simulink model "gm_lms"  (R2024a)
settings: Solver=FixedStepDiscrete  StartTime=0.0  StopTime=(samples-1)/fs  RelTol=1e-3  EnableMultiTasking=on
InitFcn:
  | setup;
undefined symbols (not defined in the file or in its folder): fs
libraries: dspadpt3 x1, dspsrcs4 x1
settings Model: Creator=ross  LastModifiedBy=ADMIN
settings SolverCC: AlgebraicLoopSolver=TrustRegion
settings DataIOCC: LimitDataPoints=on  SaveFormat=Array  SignalLogging=off  ReturnWorkspaceOutputs=off
settings OptimizationCC: BlockReduction=off  ConditionallyExecuteInputs=off  DefaultParameterBehavior=Inlined  LifeSpan=inf
settings DebuggingCC: AlgebraicLoopMsg=error  UnderspecifiedInitializationDetection=Classic  MergeDetectMultiDrivingBlocksExec=none  SolverPrmCheckMsg=warning  InheritedTsInSrcMsg=none  Int32ToFloatConvMsg=none  UnconnectedInputMsg=warning  UnconnectedOutputMsg=warning  UnconnectedLineMsg=warning  StateNameClashWarn=warning  SFUnexpectedBacktrackingDiag=warning  SFNoUnconditionalDefaultTransitionDiag=warning  SFExecutionAtInitializationDiag=none  ArithmeticOperatorsInVariantConditions=warning
settings HardwareCC: ProdBitPerPointer=32  ProdBitPerSizeT=32  ProdBitPerPtrDiffT=32  ProdLargestAtomicFloat=None  ProdIntDivRoundTo=Undefined  ProdEndianess=Unspecified  ProdWordSize=32  ProdHWDeviceType=ASIC/FPGA->ASIC/FPGA  ProdEqTarget=off
settings ModelReferenceCC: PropagateSignalLabelsOutOfModel=off
settings SFSimCC: SimUseLocalCustomCode=off  CustomCodeUndefinedFunction=UseInterfaceOnly
settings RTWCC: GenerateReport=on  RTWUseLocalCustomCode=off  GPUComputeCapability=3.5
settings CodeAppCC: StateflowObjectComments=on
settings GRTTargetCC: TargetLangStandard=C89/C90 (ANSI)
settings ConfigComp: CovMetricSettings=dw  CovSaveCumulativeToWorkspaceVar=on  CovSaveSingleToWorkspaceVar=on  CovExternalEMLEnable=off

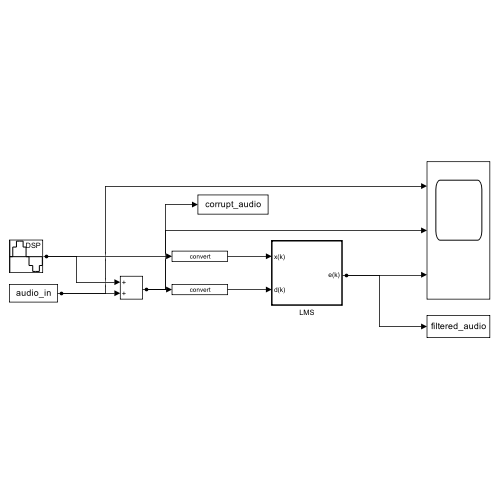
[thumbnail: Simulink's stored preview of the top-level diagram]
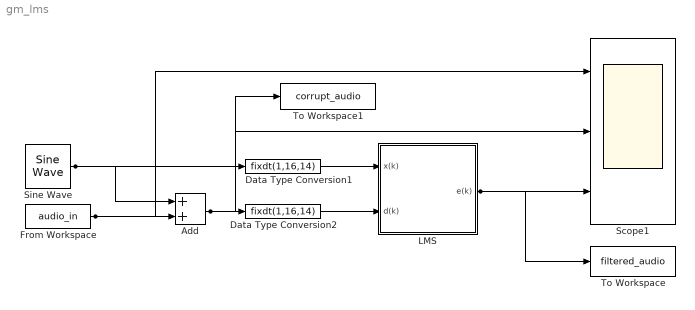
== system gm_lms ==
  Add : Sum
  Data Type Conversion1 : DataTypeConversion  OutDataTypeStr=fixdt(1,16,14)  SaturateOnIntegerOverflow=off  RndMeth=Floor
  Data Type Conversion2 : DataTypeConversion  OutDataTypeStr=fixdt(1,16,14)  SaturateOnIntegerOverflow=off  RndMeth=Floor
  From Workspace : FromWorkspace  VariableName=audio_in  SampleTime=1/fs  Interpolate=off  ZeroCross=off  OutputAfterFinalValue=Holding final value
  LMS : Subsystem  TreatAsAtomicUnit=on
  Scope1 : Scope  NumInputPorts=3
  Sine Wave : dspsrcs4/Sine Wave  Amplitude=0.75  Frequency=0.25*fs  Phase=0  SampleMode=Discrete  OutComplex=Real  CompMethod=Table lookup  TableSize=Speed  SampleTime=1/fs  SamplesPerFrame=1  ResetState=Restart at time zero  OutputFrames=on  dataType=Fixed-point  wordLen=16  udDataType=sfix(16)  fracBitsMode=User-defined  numFracBits=14  OutDataTypeStr=fixdt(1,16,14)  LastOutDataTypeStr=fixdt(1,16,14)
  To Workspace : ToWorkspace  VariableName=filtered_audio  SampleTime=-1
  To Workspace1 : ToWorkspace  VariableName=corrupt_audio  SampleTime=-1
  wires:
  Data Type Conversion2/1 -> LMS/2(d(k))
  Data Type Conversion1/1 -> LMS/1(x(k))
  LMS/1(e(k)) -> Scope1/3, To Workspace/1
  Add/1 -> Scope1/2, To Workspace1/1, Data Type Conversion2/1
  From Workspace/1 -> Add/2, Scope1/1
  Sine Wave/1 -> Data Type Conversion1/1, Add/1

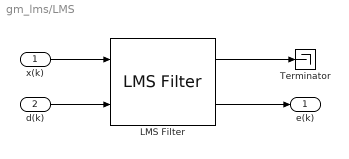
== system gm_lms/LMS ==
  x(k) : Inport
  d(k) : Inport  Port=2
  LMS Filter : dspadpt3/LMS Filter  Algo=LMS  L=16  stepflag=Dialog  mu=0.125  leakage=1.0  ic=0  Adapt=off  resetflag=None  weights=off  addnparflag=off  roundingMode=Convergent  overflowMode=off  secondCoeffMode=Binary point scaling  secondCoeffWordLength=2  secondCoeffFracLength=15  prodOutput2Mode=Binary point scaling  prodOutput2FracLength=20  prodOutput3Mode=Binary point scaling  prodOutput3FracLength=20  prodOutput4Mode=Binary point scaling  prodOutput4FracLength=20  quotientMode=Binary point scaling  quotientFracLength=20  accum2Mode=Binary point scaling  accum2FracLength=20
  Terminator : Terminator
  e(k) : Outport
  wires:
  LMS Filter/1 -> Terminator/1
  LMS Filter/2 -> e(k)/1
  x(k)/1 -> LMS Filter/1
  d(k)/1 -> LMS Filter/2
